simulink model "com_simulink_realim_estados_F"  (R2026a)
settings: Solver=VariableStepAuto  StopTime=Inf
libraries: instrumentseriallib x2, simulink x1
settings Model: Creator=Claudio  LastModifiedBy=Dante P

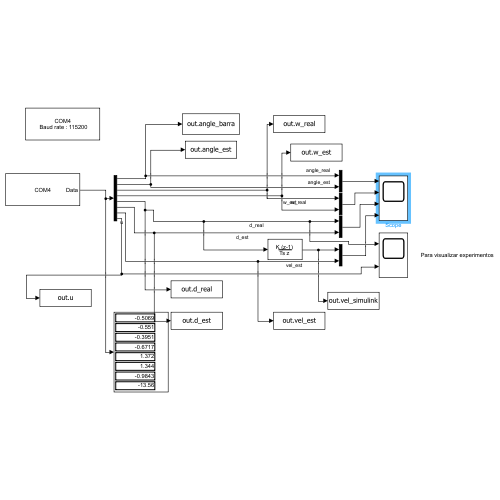
[thumbnail: Simulink's stored preview of the top-level diagram]
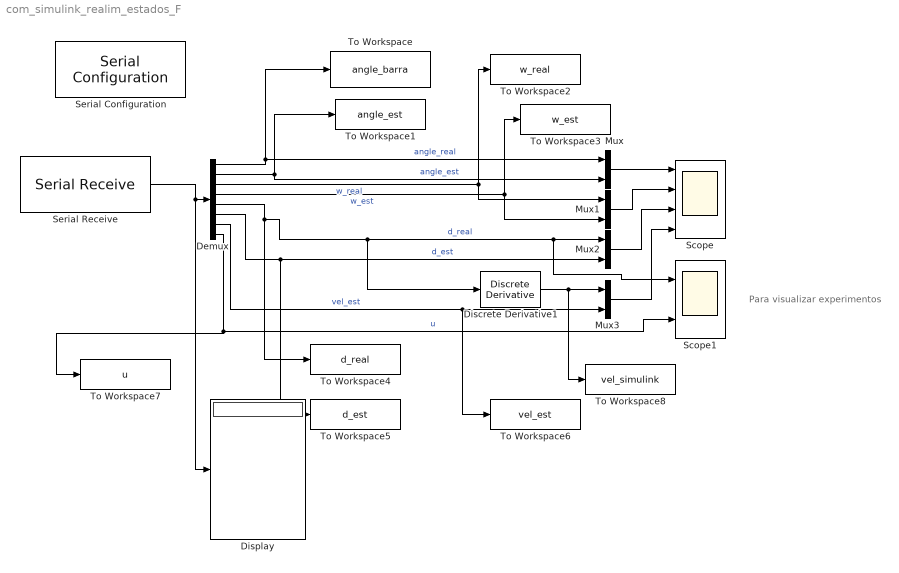
== system com_simulink_realim_estados_F ==
  note: Para visualizar experimentos
  Demux : Demux  Outputs=8
  Discrete Derivative1 : simulink/Discrete/Discrete Derivative  gainval=1.0  ICPrevScaledInput=-580  OutMin=[]  OutMax=[]  OutDataType=fixdt(1, 16)  OutScaling=2^-10  DoSatur=off
  Display : Display
  Mux{,1..3} (4 alike) : Mux  Inputs=2
  Scope : Scope  NumInputPorts=4
      settings: TimeSpan=60  ActiveDisplayString=4  ActiveDisplayYMinimum=-115.22259712219237  ActiveDisplayYMaximum=763.84526252746582
  Scope1 : Scope  NumInputPorts=2
      settings: TimeSpan=60  ActiveDisplayYMinimum=-12.037935376167297  ActiveDisplayYMaximum=1.1931906938552854
  Serial Configuration : instrumentseriallib/Serial Configuration  Priority=-200000  PortSel=COM4  Port=COM4  ComPort=COM4  BaudRate=115200  DataBits=8  Parity=none  StopBits=1  ByteOrder=big-endian  FlowControl=none  Timeout=10  SimulateUsing=Interpreted execution  BlockInModel=on  aMode=1
  Serial Receive : instrumentseriallib/Serial Receive  Priority=1  PortSel=COM4  Port=COM4  ComPort=COM4  DataType=single  SaveDataType=uint8  ToggleHeader=on  Header="[ 97   98   99  100 ]"  ToggleDataSize=on  DataSize=[8 1]  ToggleTerminator=off  Terminator=<none>  CustomTerminator=[]  InputFormat=Column major  EnableBlockingMode=on  ActionDataUnavailable=Output last received value  ActionWhenDataUnavailable=Output last received value  CustomValue=0  SampleTime=0.02  SimulateUsing=Interpreted execution  BlockInModel=on  aMode=1  LibraryInUse=instrumentlib
  To Workspace : ToWorkspace  VariableName=angle_barra  SampleTime=-1
      settings: Save2DSignal=2-D array (concatenate along first dimension)
  To Workspace1 : ToWorkspace  VariableName=angle_est  SampleTime=-1
      settings: Save2DSignal=2-D array (concatenate along first dimension)
  To Workspace2 : ToWorkspace  VariableName=w_real  SampleTime=-1
      settings: Save2DSignal=2-D array (concatenate along first dimension)
  To Workspace3 : ToWorkspace  VariableName=w_est  SampleTime=-1
      settings: Save2DSignal=2-D array (concatenate along first dimension)
  To Workspace4 : ToWorkspace  VariableName=d_real  SampleTime=-1
      settings: Save2DSignal=2-D array (concatenate along first dimension)
  To Workspace5 : ToWorkspace  VariableName=d_est  SampleTime=-1
      settings: Save2DSignal=2-D array (concatenate along first dimension)
  To Workspace6 : ToWorkspace  VariableName=vel_est  SampleTime=-1
      settings: Save2DSignal=2-D array (concatenate along first dimension)
  To Workspace7 : ToWorkspace  VariableName=u  SampleTime=-1
      settings: Save2DSignal=2-D array (concatenate along first dimension)
  To Workspace8 : ToWorkspace  VariableName=vel_simulink  SampleTime=-1
      settings: Save2DSignal=2-D array (concatenate along first dimension)
  wires:
  Demux/2 -> To Workspace1/1, Mux/2  "angle_est"
  Demux/1 -> To Workspace/1, Mux/1  "angle_real"
  Serial Receive/1 -> Display/1, Demux/1
  Demux/3 -> Mux1/1, To Workspace2/1  "w_real"
  Demux/4 -> Mux1/2, To Workspace3/1  "w_est"
  Mux/1 -> Scope/1
  Mux1/1 -> Scope/2
  Mux2/1 -> Scope/3
  Demux/5 -> To Workspace4/1, Discrete Derivative1/1, Scope1/1, Mux2/1  "d_real"
  Demux/6 -> To Workspace5/1, Mux2/2  "d_est"
  Demux/7 -> Mux3/2, To Workspace6/1  "vel_est"
  Demux/8 -> Scope1/2, To Workspace7/1  "u"
  Mux3/1 -> Scope/4
  Discrete Derivative1/1 -> To Workspace8/1, Mux3/1
